simulink model "speed_current_mech"  (R2024a)
settings: Solver=FixedStepAuto  StartTime=0.0  StopTime=3  FixedStep=1e-6  RelTol=1e-6
values from neighbouring files (symbols this model uses):
  B = 0.001    [main.m]
  Ia_rated = 30    [main.m]
  J = 0.003    [main.m]
  Kac = 1/Kpc    (= 1.59154943092)    [main.m]
  Ke = Kt    (= 0.318309886184)    [main.m]
  Kic = Ra * Wcc    (= 94.2477796077)    [main.m]
  Kis = J*Wsc^2/(5*Kt)    (= 7.44150640327)    [main.m]
  Kpc = La * Wcc    (= 0.628318530718)    [main.m]
  Kps = J*Wsc/Kt    (= 0.592176264065)    [main.m]
  Kt = Te_rated/Ia_rated    (= 0.318309886184)    [main.m]
  La = 2.0e-3    (= 0.002)    [main.m]
  Ra = 0.3    [main.m]
  TL = 8.5    [main.m]
  Tsw = 1/Fsw    (= 0.0005)    [main.m]
  Va_rated = 100    [main.m]
  Vdc = 150    [main.m]
libraries: simulink x1
settings Model: Creator=moon  LastModifiedBy=moon

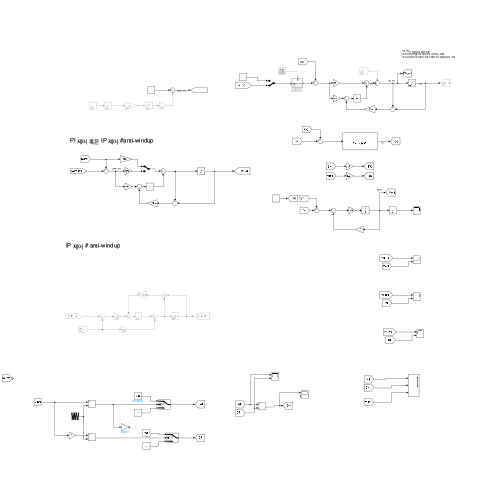
[thumbnail: Simulink's stored preview of the top-level diagram]
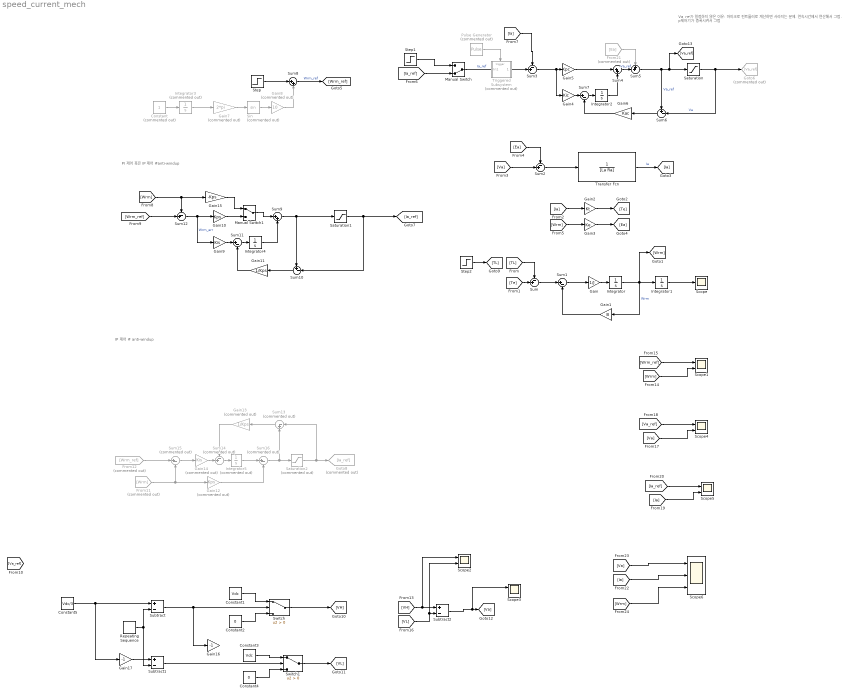
== system speed_current_mech ==
  note: Va_ref가 일정하지 않은 이유:
      | 마이크로 컨트롤러로 계산하면 사라지는 문제.
      | 연속시간에서 연산해서 그럼. p제어기가 증폭시켜서 그럼
  note: PI 제어 혹은 IP 제어 #anti-windup
  note: IP 제어 # anti-windup
  Constant : Constant  Commented=on
  Constant1 : Constant  Value=Vdc
  Constant2 : Constant  Value=0
  Constant3 : Constant  Value=Vdc
  Constant4 : Constant  Value=0
  Constant5 : Constant  Value=Vdc/3
  From11 : From  Commented=on  GotoTag=Wrm
  From12 : From  Commented=on  GotoTag=Wrm_ref
  From21 : From  Commented=on  GotoTag=Ea
  Gain : Gain  Gain=1/J
  Gain1 : Gain  Gain=B
  Gain10 : Gain  Gain=Kps
  Gain11 : Gain  Gain=1/Kps
  Gain12 : Gain  Commented=on  Gain=Kps
  Gain13 : Gain  Commented=on  Gain=1/Kps
  Gain14 : Gain  Commented=on  Gain=Kis
  Gain15 : Gain  Gain=-Kps
  Gain16 : Gain  Gain=-1
  Gain17 : Gain  Gain=-1
  Gain2 : Gain  Gain=Kt
  Gain3 : Gain  Gain=Ke
  Gain4 : Gain  Gain=Kic
  Gain5 : Gain  Gain=Kpc
  Gain6 : Gain  Gain=Kac
  Gain7 : Gain  Commented=on  Gain=2*pi
  Gain8 : Gain  Commented=on  Gain=10
  Gain9 : Gain  Gain=Kis
  Goto6 : Goto  Commented=on  GotoTag=Va_ref
  Goto8 : Goto  Commented=on  GotoTag=Ia_ref
  Integrator{,1..2,4} (4 alike) : Integrator
  Integrator3 : Integrator  Commented=on
  Integrator5 : Integrator  Commented=on
  Manual Switch : ManualSwitch  CurrentSetting=0
  Manual Switch1 : ManualSwitch
  Pulse Generator : DiscretePulseGenerator  Commented=on  PulseType=Time based  Period=Tsw  PulseWidth=5
  Repeating Sequence : simulink/Sources/Repeating Sequence  rep_seq_t=[0 Tsw/2 Tsw]  rep_seq_y=[Vdc -Vdc Vdc]
  Saturation : Saturate  UpperLimit=Va_rated  LowerLimit=-Va_rated
  Saturation1 : Saturate  UpperLimit=Ia_rated  LowerLimit=-Ia_rated
  Saturation2 : Saturate  Commented=on  UpperLimit=Ia_rated  LowerLimit=-Ia_rated
  Scope : Scope
  Scope{1..5} (5 alike) : Scope  NumInputPorts=2
  Scope6 : Scope  NumInputPorts=3
  Sin : Trigonometry  Commented=on
  Step : Step  Time=0.1  After=200  SampleTime=0
  Step1 : Step  After=Ia_rated  SampleTime=0
  Step2 : Step  Time=0.3  After=TL  SampleTime=0
  Subtract : Sum  Inputs=+-
  Subtract1 : Sum  Inputs=+-
  Subtract2 : Sum  Inputs=+-
  Sum{,2..3,12} (4 alike) : Sum  Inputs=-+|
  Sum1 : Sum  Inputs=|+-
  Sum10 : Sum  Inputs=+-|
  Sum11 : Sum  Inputs=|+-
  Sum13 : Sum  Commented=on  Inputs=|-+
  Sum14 : Sum  Commented=on  Inputs=-+|
  Sum15 : Sum  Commented=on  Inputs=|+-
  Sum16 : Sum  Commented=on  Inputs=|+-
  Sum4 : Sum  Inputs=|++
  Sum5 : Sum  Inputs=++|
  Sum6 : Sum  Inputs=+-|
  Sum7 : Sum  Inputs=|+-
  Sum8 : Sum  Inputs=|++
  Sum9 : Sum  Inputs=|++
  Switch : Switch  Criteria=u2 > Threshold  SaturateOnIntegerOverflow=off  InputSameDT=off
  Switch1 : Switch  Criteria=u2 > Threshold  SaturateOnIntegerOverflow=off  InputSameDT=off
  Transfer Fcn : TransferFcn  Denominator=[La Ra]
  Triggered Subsystem : Subsystem  Commented=on  TreatAsAtomicUnit=on
  wires:
  [Te] -> Sum/2
  [TL] -> Sum/1
  Sum/1 -> Sum1/1
  Sum1/1 -> Gain/1
  Gain/1 -> Integrator/1
  Gain1/1 -> Sum1/2
  Integrator/1 -> [Wrm], Integrator1/1, Gain1/1  "Wrm"
  Integrator1/1 -> Scope/1
  [Ia] -> Gain2/1
  Gain2/1 -> [Te]
  Transfer Fcn/1 -> [Ia]  "Ia"
  [Va] -> Sum2/2
  Sum2/1 -> Transfer Fcn/1
  [Ea] -> Sum2/1
  Gain3/1 -> [Ea]
  [Wrm] -> Gain3/1
  Manual Switch/1 -> Sum3/2  "Ia_ref"
  [Ia] -> Sum3/1
  Sum3/1 -> Gain5/1, Gain4/1
  Sum5/1 -> Sum6/1, [Va_ref], Saturation/1  "Va_ref"
  Saturation/1 -> Sum6/2, Goto6/1  "Va"
  Sum6/1 -> Gain6/1
  Integrator2/1 -> Sum4/2
  Gain5/1 -> Sum4/1
  Gain4/1 -> Sum7/1
  Sum7/1 -> Integrator2/1
  Gain6/1 -> Sum7/2
  Step/1 -> Sum8/1
  Constant/1 -> Integrator3/1
  Integrator3/1 -> Gain7/1
  Gain7/1 -> Sin/1
  Sin/1 -> Gain8/1
  Gain8/1 -> Sum8/2
  Sum8/1 -> [Wrm_ref]  "Wrm_ref"
  Sum12/1 -> Gain10/1, Gain9/1  "Wrm_err"
  Integrator4/1 -> Sum9/2
  Sum9/1 -> Saturation1/1, Sum10/1
  Step1/1 -> Manual Switch/1
  [Ia_ref] -> Manual Switch/2
  Sum10/1 -> Gain11/1
  Gain9/1 -> Sum11/1
  Sum11/1 -> Integrator4/1
  Gain11/1 -> Sum11/2
  Saturation1/1 -> Sum10/2, [Ia_ref]
  Sum16/1 -> Sum13/2, Saturation2/1
  Sum15/1 -> Gain14/1
  Saturation2/1 -> Sum13/1, Goto8/1
  From12/1 -> Sum15/1
  Integrator5/1 -> Sum16/1
  Gain12/1 -> Sum16/2
  From11/1 -> Gain12/1, Sum15/2
  Sum13/1 -> Gain13/1
  Gain14/1 -> Sum14/2
  Sum14/1 -> Integrator5/1
  Gain13/1 -> Sum14/1
  Step2/1 -> [TL]
  [Wrm_ref] -> Scope1/1
  [Wrm] -> Scope1/2
  [Wrm] -> Sum12/1, Gain15/1
  Gain15/1 -> Manual Switch1/1
  Gain10/1 -> Manual Switch1/2
  Manual Switch1/1 -> Sum9/1
  [Wrm_ref] -> Sum12/2
  Repeating Sequence/1 -> Subtract1/2, Subtract/2
  Gain17/1 -> Subtract1/1
  Constant1/1 -> Switch/1
  Constant2/1 -> Switch/3
  Subtract/1 -> Gain16/1, Switch/2
  Constant3/1 -> Switch1/1
  Constant4/1 -> Switch1/3
  Subtract1/1 -> Switch1/2
  Switch/1 -> [VH]
  Switch1/1 -> [VL]
  [VH] -> Scope2/1, Subtract2/1
  [VL] -> Subtract2/2, Scope2/2
  Subtract2/1 -> Scope3/1, [Va]
  [Va_ref] -> Scope4/1
  [Va] -> Scope4/2
  [Ia_ref] -> Scope5/1
  [Ia] -> Scope5/2
  Pulse Generator/1 -> Triggered Subsystem/Trigger
  From21/1 -> Sum5/1
  Sum4/1 -> Sum5/2  "Va_ref"
  [Va] -> Scope6/1
  [Ia] -> Scope6/2
  [Wrm] -> Scope6/3
  Constant5/1 -> Gain17/1, Subtract/1

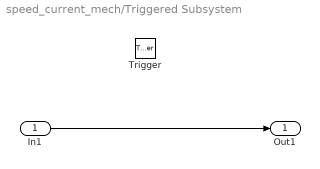
== system speed_current_mech/Triggered Subsystem ==
  In1 : Inport
  Trigger : TriggerPort  VariantControl=(inherit)
  Out1 : Outport
  wires:
  In1/1 -> Out1/1
